simulink model "HILsim"  (R2024a)
settings: Solver=ode8  StartTime=0.0  StopTime=inf  FixedStep=SampleTime  RelTol=1e-3
values from neighbouring files (symbols this model uses):
  Arm = [ ... (first row only)    [launch.m]
  CDDrone = 0.01    [launch.m]
  CDval = 0.008    [launch.m]
  g = 9.81    [launch.m]
  m = 1.9    [launch.m]
  m_to_mm = 1000    [launch.m]
  ms_to_cms = 100    [launch.m]
  prop_inertia = (1/12) * 0.015 * 0.127^2    (= 2.016125e-05)    [launch.m]
  R = 0.127    [launch.m]
  ref_height = 76    [launch.m]
  ref_lat = 437818446e-7    (= 43.7818446)    [launch.m]
  ref_lon = -794679715e-7    (= -79.4679715)    [launch.m]
  rotorRPMMax = 10000    [launch.m]
  rotorTimeConst = 0.05    [launch.m]
  SampleTime = 0.004    [launch.m]
  tilt_speed = [0; pi/4; 0]    [launch.m]
  uT_to_gauss = 0.01    [launch.m]
undefined symbols (not defined in the file or in its folder): contact, control, ddx, ddy, ddz, dx, dy, dz, fractalcoef, lastVh, p, Payload, pitch, q, r, roll, X, Y, yaw, Z
libraries: uavmavlinklib x9, simulink x3, sharedutil x3, px4MAVLinkBridgelib x2, aerolibatmos2 x1, sensorgpslib x1, robotcorelib x1, mspsensorlib x1, shared6dof x1, simulink_extras x1, matrix_library x1
(part 2 of 2)

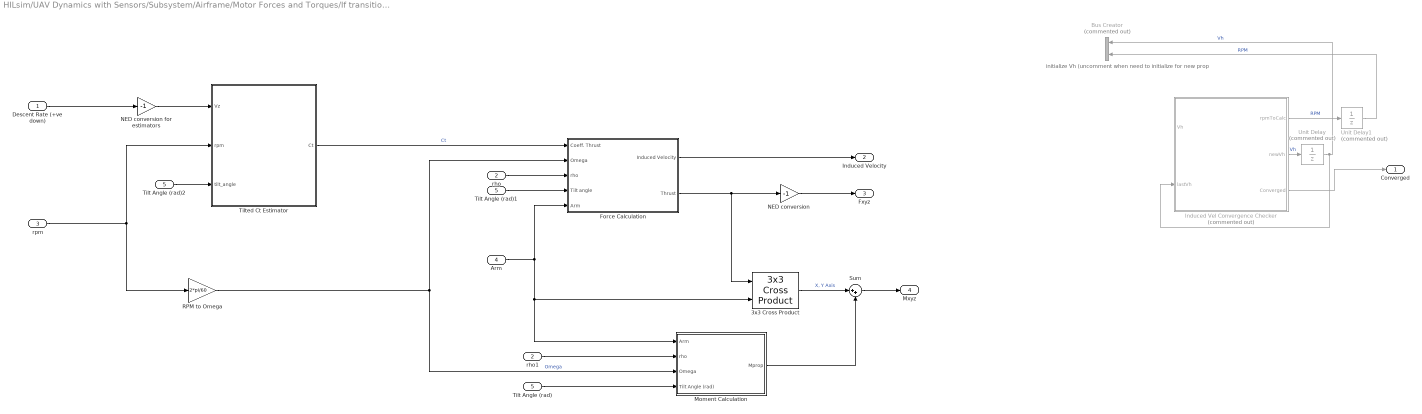
== system HILsim/UAV Dynamics with Sensors/Subsystem/Airframe/Motor Forces and Torques/If transitioning/Multirotor Subsystem/Rotor Subsystem ==
  note: initialize Vh (uncomment when need to initialize for new prop
  Descent Rate (+ve down) : Inport
  rho : Inport  Port=2
  rpm : Inport  Port=3
  Arm : Inport  Port=4
  Tilt Angle (rad) : Inport  Port=5
  3x3 Cross Product : sharedutil/3x3 Cross Product  aMode=aMode
      settings: LibrarySourceBlock=aerolibutil/3x3 Cross Product
  Bus Creator : BusCreator  Commented=on  Inputs=2
  Force Calculation : Subsystem
  Induced Vel Convergence Checker : MATLAB Function  Commented=on  TreatAsAtomicUnit=on  mask{VhInit=4.7, ConvThresh=1e-4}
      mask prompts: VhInit "Initial Vh Guess"; ConvThresh "Convergence Threshold"
  Moment Calculation : Subsystem
  NED conversion : Gain  Gain=-1
  NED conversion for estimators : Gain  Gain=-1
  RPM to Omega : Gain  Gain=2*pi/60
  Sum : Sum  Inputs=|++
  Tilt Angle (rad)1 : InportShadow  Port=5
  Tilt Angle (rad)2 : InportShadow  Port=5
  Tilted Ct Estimator : Subsystem
  Unit Delay : UnitDelay  Commented=on  InitialCondition=lastVh  SampleTime=0.001  HasFrameUpgradeWarning=on
  Unit Delay1 : UnitDelay  Commented=on  InitialCondition=1  SampleTime=0.001  HasFrameUpgradeWarning=on
  rho1 : InportShadow  Port=2
  Converged : Outport
  Induced Velocity : Outport  Port=2
  Fxyz : Outport  Port=3
  Mxyz : Outport  Port=4
  wires:
  Tilted Ct Estimator/1(Ct) -> Force Calculation/1(Coeff. Thrust)  "Ct"
  Unit Delay/1 -> Bus Creator/1, Induced Vel Convergence Checker/2(lastVh)  "Vh"
  Induced Vel Convergence Checker/3(Converged) -> Converged/1
  RPM to Omega/1 -> Moment Calculation/3(Omega), Force Calculation/2(Omega)  "Omega"
  rho/1 -> Force Calculation/3(rho)
  Induced Vel Convergence Checker/2(newVh) -> Unit Delay/1  "Vh"
  rpm/1 -> RPM to Omega/1, Tilted Ct Estimator/2(rpm)
  Descent Rate (+ve down)/1 -> NED conversion for estimators/1
  Unit Delay1/1 -> Bus Creator/2  "RPM"
  Induced Vel Convergence Checker/1(rpmToCalc) -> Unit Delay1/1  "RPM"
  Force Calculation/1(Induced Velocity) -> Induced Velocity/1
  Force Calculation/2(Thrust) -> NED conversion/1, 3x3 Cross Product/1
  3x3 Cross Product/1 -> Sum/1  "X, Y Axis"
  rho1/1 -> Moment Calculation/2(rho)
  Arm/1 -> 3x3 Cross Product/2, Moment Calculation/1(Arm), Force Calculation/5(Arm)
  Moment Calculation/1(Mprop) -> Sum/2
  Sum/1 -> Mxyz/1
  NED conversion/1 -> Fxyz/1
  Tilt Angle (rad)/1 -> Moment Calculation/4(Tilt Angle (rad))
  Tilt Angle (rad)1/1 -> Force Calculation/4(Tilt angle)
  NED conversion for estimators/1 -> Tilted Ct Estimator/1(Vz)
  Tilt Angle (rad)2/1 -> Tilted Ct Estimator/3(tilt_angle)

== system HILsim/UAV Dynamics with Sensors/Subsystem/Airframe/Motor Forces and Torques/If Tilted/Multirotor Subsystem/Rotor Subsystem/Ct Estimator ==
  note: this Vh curve is derived from performing a convergence
      | on the thrust curve
  note: Ct and Ct/Ct0 estimators are derived from CFD data
  Vz : Inport
  rpm : Inport  Port=2
  Abs : Abs  SaturateOnIntegerOverflow=off
  Calculate Ct : Product  Inputs=**
  Ct/C0 State Switcher : Subsystem
  Ct/Ct0 Estimator : Polyval  Coefs=[-0.012716815691322, -0.022830541813396, 0.156313447084851, -0.031641009616291, 1.004637965110952]
  Ct0 estimator for RPM : Polyval  Coefs=[0.000000000012185, -0.000000274732884, 0.008305365728125]
  Divide1 : Product  Inputs=*/
  NED conversion for estimators : Gain  Gain=-1
  Vh Calculator : Polyval  Coefs=[-5.17622414362771e-09, 0.000822973507549008, 0.0232660553338375]
  Ct : Outport
  wires:
  Abs/1 -> Ct0 estimator for RPM/1, Vh Calculator/1
  Divide1/1 -> Ct/Ct0 Estimator/1, Ct/C0 State Switcher/1(" Vz/Vh")  "Vz/Vh"
  Vh Calculator/1 -> Divide1/2  "Vh"
  Ct0 estimator for RPM/1 -> Calculate Ct/2  "Ct0"
  NED conversion for estimators/1 -> Divide1/1
  Ct/Ct0 Estimator/1 -> Ct/C0 State Switcher/2(Ct/C0 Fit)  "Ct/C0 Fit"
  Ct/C0 State Switcher/1(Out1) -> Calculate Ct/1  "Ct/C0"
  rpm/1 -> Abs/1
  Vz/1 -> NED conversion for estimators/1
  Calculate Ct/1 -> Ct/1  "Ct"

== system HILsim/UAV Dynamics with Sensors/Subsystem/Airframe/Motor Forces and Torques/If Tilted/Multirotor Subsystem/Rotor Subsystem/Force Calculation ==
  Coeff. Thrust : Inport
  Omega : Inport  Port=2
  rho : Inport  Port=3
  Arm : Inport  Port=4
  Constant : Constant  Value=0
  Divide : Product  Inputs=**
  Fx Sign : Subsystem
  Gain : Gain  Gain=cos(pi/4)
  Gain1 : Gain  Gain=sin(pi/4)
  Induced Vel Calc : Subsystem
  Math Function3 : Math  Operator=square  SignedPower=on
  Mux : Mux  Inputs=3
  Product6 : Product  Inputs=3
  R3 : Gain  Gain=R*R*pi*R*R
  Induced Velocity : Outport
  Thrust : Outport  Port=2
  wires:
  Math Function3/1 -> R3/1
  Induced Vel Calc/1(Vh) -> Induced Velocity/1
  R3/1 -> Product6/2
  Omega/1 -> Math Function3/1
  Gain1/1 -> Mux/3  "Fz"
  Constant/1 -> Mux/2  "Fy"
  Divide/1 -> Gain/1
  Product6/1 -> Divide/2, Gain1/1, Induced Vel Calc/1(Thrust)  "Fx"
  Fx Sign/1(Xsign) -> Divide/1
  Arm/1 -> Fx Sign/1(Arm)
  Gain/1 -> Mux/1  "Fx"
  Mux/1 -> Thrust/1
  Coeff. Thrust/1 -> Product6/3
  rho/1 -> Product6/1

== system HILsim/UAV Dynamics with Sensors/Subsystem/Airframe/Motor Forces and Torques/If Tilted/Multirotor Subsystem/Rotor Subsystem/Moment Calculation ==
  note: $\text{Torque about }z\text{ axis for the }i\text{th motor}: \frac{-1}{\sqrt2}(b\omega^2 + I_M \dot{w}), \text{where } b = \rho C_D AR^3$
  note: Angular Acceleration Term - $I_m \dot{\omega}$
  Arm : Inport
  rho : Inport  Port=2
  Omega : Inport  Port=3
  Abs : Abs  SaturateOnIntegerOverflow=off
  Divide : Product  Inputs=**
  Matrix Multiply : Product
  Moment of Inertia (1/12 m (a^2 + b^2)) : Gain  Gain=prop_inertia
  Mx Sign : Subsystem
  Mxy : Constant  Value=[0]
  OmegaDot : Derivative
  Product7 : Product
  R4 : Gain  Gain=CDval*R*R*R*pi*R*R
  Sum : Sum  Inputs=|++
  Vector Concatenate3 : Concatenate  NumInputs=3
  X : Gain  Gain=-1/sqrt(2)
  Z : Gain  Gain=-1/sqrt(2)
  Mprop : Outport
  wires:
  Vector Concatenate3/1 -> Mprop/1
  Omega/1 -> Abs/1, OmegaDot/1, Matrix Multiply/1
  OmegaDot/1 -> Moment of Inertia (1/12 m (a^2 + b^2))/1  "OmegaDot"
  Sum/1 -> Z/1, Divide/2
  Product7/1 -> Sum/1
  Moment of Inertia (1/12 m (a^2 + b^2))/1 -> Sum/2
  Z/1 -> Vector Concatenate3/3
  Divide/1 -> X/1
  Mxy/1 -> Vector Concatenate3/2  "Y"
  X/1 -> Vector Concatenate3/1
  Arm/1 -> Mx Sign/1(Arm)
  Mx Sign/1(Xsign) -> Divide/1
  Matrix Multiply/1 -> R4/1
  Abs/1 -> Matrix Multiply/2
  rho/1 -> Product7/1
  R4/1 -> Product7/2

== system HILsim/UAV Dynamics with Sensors/Subsystem/Airframe/Motor Forces and Torques/If non tilted/Multirotor Subsystem/Rotor Subsystem/Force Calculation ==
  Coeff. Thrust : Inport
  Omega : Inport  Port=2
  rho : Inport  Port=3
  Constant : Constant  Value=[0;0]  VectorParams1D=off
  Induced Vel Calc : Subsystem
  Math Function3 : Math  Operator=square  SignedPower=on
  Product6 : Product  Inputs=3
  R3 : Gain  Gain=R*R*pi*R*R
  Vector Concatenate : Concatenate
  Induced Velocity : Outport
  Thrust : Outport  Port=2
  wires:
  Coeff. Thrust/1 -> Product6/1
  Math Function3/1 -> R3/1
  Induced Vel Calc/1(Vh) -> Induced Velocity/1
  R3/1 -> Product6/2
  rho/1 -> Product6/3
  Omega/1 -> Math Function3/1
  Product6/1 -> Vector Concatenate/2, Induced Vel Calc/1(Thrust)  "Fz"
  Vector Concatenate/1 -> Thrust/1
  Constant/1 -> Vector Concatenate/1

== system HILsim/UAV Dynamics with Sensors/Subsystem/Airframe/Motor Forces and Torques/If non tilted/Multirotor Subsystem/Rotor Subsystem/Moment Calculation ==
  note: $\text{Torque about }z\text{ axis for the }i\text{th motor}: \frac{-1}{\sqrt2}(b\omega^2 + I_M \dot{w}), \text{where } b = \rho C_D AR^3$
  note: Angular Acceleration Term - $I_m \dot{\omega}$
  rho : Inport
  Omega : Inport  Port=2
  Abs : Abs  SaturateOnIntegerOverflow=off
  Matrix Multiply : Product
  Moment of Inertia (1/12 m (a^2 + b^2)) : Gain  Gain=prop_inertia
  Mxy : Constant  Value=[0;0]  VectorParams1D=off
  OmegaDot : Derivative
  Product7 : Product
  R4 : Gain  Gain=CDval*R*R*R*pi*R*R
  Sum : Sum  Inputs=|++
  Vector Concatenate3 : Concatenate
  Z : Gain  Gain=-1/sqrt(2)
  Mprop : Outport
  wires:
  Vector Concatenate3/1 -> Mprop/1
  R4/1 -> Product7/2
  rho/1 -> Product7/1
  Omega/1 -> Abs/1, OmegaDot/1, Matrix Multiply/1
  OmegaDot/1 -> Moment of Inertia (1/12 m (a^2 + b^2))/1  "OmegaDot"
  Sum/1 -> Z/1
  Product7/1 -> Sum/1
  Moment of Inertia (1/12 m (a^2 + b^2))/1 -> Sum/2
  Z/1 -> Vector Concatenate3/2
  Matrix Multiply/1 -> R4/1
  Abs/1 -> Matrix Multiply/2
  Mxy/1 -> Vector Concatenate3/1  "XY"

== system HILsim/UAV Dynamics with Sensors/Subsystem/Airframe/Motor Forces and Torques/If non tilted/Multirotor Subsystem/Rotor Subsystem/Non Tilted Ct estimator ==
  Vz : Inport
  RPM : Inport  Port=2
  Abs : Abs  SaturateOnIntegerOverflow=off
  Calculate Ct : Product  Inputs=**
  Ct/C0 State Switcher : Subsystem
  Ct/Ct0 Non Tilted Estimator : Polyval  Coefs=[0.147117704259973, 0.135195473604728, -0.341999514591595, -0.246799876690693, 0.999678014049876]
  Ct0 estimator for RPM : Polyval  Coefs=[0.000000000012185, -0.000000274732884, 0.008305365728125]
  Divide1 : Product  Inputs=*/
  Vh Calculator : Polyval  Coefs=[-5.17622414362771e-09, 0.000822973507549008, 0.0232660553338375]
  Ct : Outport
  wires:
  Abs/1 -> Vh Calculator/1, Ct0 estimator for RPM/1
  Calculate Ct/1 -> Ct/1  "Ct"
  Divide1/1 -> Ct/Ct0 Non Tilted Estimator/1, Ct/C0 State Switcher/1(" Vz/Vh")  "Vz/Vh"
  RPM/1 -> Abs/1
  Vh Calculator/1 -> Divide1/2  "Vh"
  Ct0 estimator for RPM/1 -> Calculate Ct/2  "Ct0"
  Ct/Ct0 Non Tilted Estimator/1 -> Ct/C0 State Switcher/2(Ct/C0 Fit)  "Ct/C0 Fit"
  Vz/1 -> Divide1/1
  Ct/C0 State Switcher/1(Ct/Ct0) -> Calculate Ct/1

== system HILsim/UAV Dynamics with Sensors/Subsystem/Airframe/Motor Forces and Torques/If transitioning/Multirotor Subsystem/Rotor Subsystem/Force Calculation ==
  Coeff. Thrust : Inport
  Omega : Inport  Port=2
  rho : Inport  Port=3
  Tilt angle : Inport  Port=4
  Arm : Inport  Port=5
  Components : Subsystem
  Fx Sign : Subsystem
  Induced Vel Calc : Subsystem
  Math Function3 : Math  Operator=square  SignedPower=on
  Mux : Mux  Inputs=3
  Product6 : Product  Inputs=3
  R3 : Gain  Gain=R*R*pi*R*R
  Induced Velocity : Outport
  Thrust : Outport  Port=2
  wires:
  Coeff. Thrust/1 -> Product6/1
  Math Function3/1 -> R3/1
  Induced Vel Calc/1(Vh) -> Induced Velocity/1
  R3/1 -> Product6/2
  rho/1 -> Product6/3
  Omega/1 -> Math Function3/1
  Product6/1 -> Components/3(F), Induced Vel Calc/1(Thrust)  "F"
  Arm/1 -> Fx Sign/1(Arm)
  Mux/1 -> Thrust/1
  Fx Sign/1(Xsign) -> Components/1(Sign)
  Tilt angle/1 -> Components/2(Tilt angle)
  Components/1(Fx) -> Mux/1
  Components/2(Fy) -> Mux/2
  Components/3(Fz) -> Mux/3

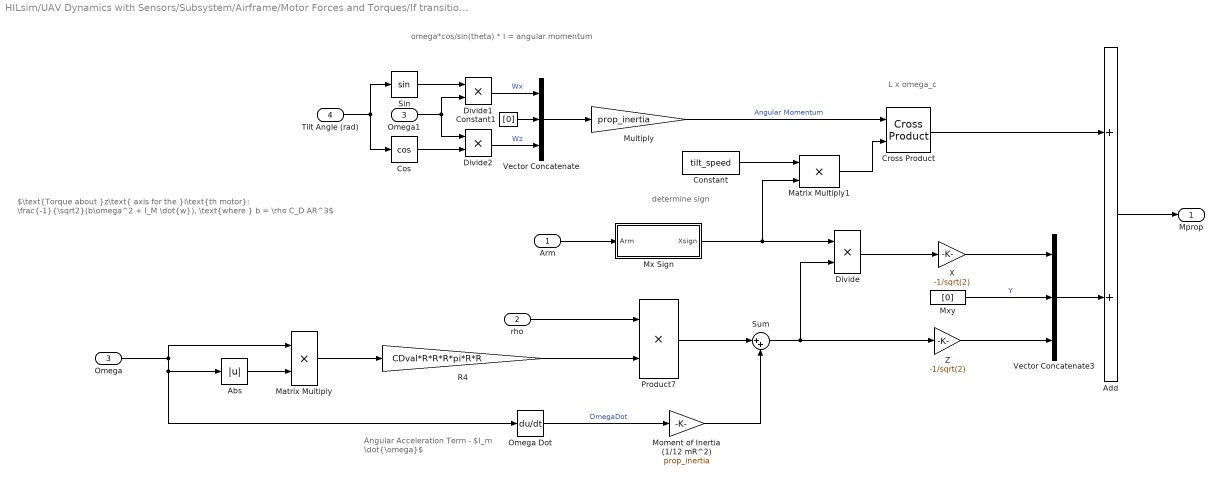
== system HILsim/UAV Dynamics with Sensors/Subsystem/Airframe/Motor Forces and Torques/If transitioning/Multirotor Subsystem/Rotor Subsystem/Moment Calculation ==
  note: determine sign
  note: L x omega_c
  note: omega*cos/sin(theta) * I = angular momentum
  note: $\text{Torque about }z\text{ axis for the }i\text{th motor}: \frac{-1}{\sqrt2}(b\omega^2 + I_M \dot{w}), \text{where } b = \rho C_D AR^3$
  note: Angular Acceleration Term - $I_m \dot{\omega}$
  Arm : Inport
  rho : Inport  Port=2
  Omega : Inport  Port=3
  Tilt Angle (rad) : Inport  Port=4
  Abs : Abs  SaturateOnIntegerOverflow=off
  Add : Sum
  Constant : Constant  Value=tilt_speed
  Constant1 : Constant  Value=[0]
  Cos : Trigonometry  Operator=cos
  Cross Product : matrix_library/Cross Product
  Divide : Product  Inputs=**
  Divide1 : Product  Inputs=**
  Divide2 : Product  Inputs=**
  Matrix Multiply : Product
  Matrix Multiply1 : Product
  Moment of Inertia (1/12 mR^2) : Gain  Gain=prop_inertia
  Multiply : Gain  Gain=prop_inertia
  Mx Sign : Subsystem
  Mxy : Constant  Value=[0]
  Omega Dot : Derivative
  Omega1 : InportShadow  Port=3
  Product7 : Product
  R4 : Gain  Gain=CDval*R*R*R*pi*R*R
  Sin : Trigonometry
  Sum : Sum  Inputs=|++
  Vector Concatenate : Concatenate  NumInputs=3
  Vector Concatenate3 : Concatenate  NumInputs=3
  X : Gain  Gain=-1/sqrt(2)
  Z : Gain  Gain=-1/sqrt(2)
  Mprop : Outport
  wires:
  R4/1 -> Product7/2
  rho/1 -> Product7/1
  Omega/1 -> Omega Dot/1, Abs/1, Matrix Multiply/1
  Omega Dot/1 -> Moment of Inertia (1/12 mR^2)/1  "OmegaDot"
  Sum/1 -> Z/1, Divide/2
  Product7/1 -> Sum/1
  Moment of Inertia (1/12 mR^2)/1 -> Sum/2
  Z/1 -> Vector Concatenate3/3
  Divide/1 -> X/1
  Mxy/1 -> Vector Concatenate3/2  "Y"
  Arm/1 -> Mx Sign/1(Arm)
  Mx Sign/1(Xsign) -> Divide/1, Matrix Multiply1/2
  Matrix Multiply/1 -> R4/1
  Abs/1 -> Matrix Multiply/2
  Tilt Angle (rad)/1 -> Cos/1, Sin/1
  Cos/1 -> Divide2/2
  Sin/1 -> Divide1/1
  Divide1/1 -> Vector Concatenate/1  "Wx"
  Vector Concatenate/1 -> Multiply/1
  Multiply/1 -> Cross Product/1  "Angular Momentum"
  Cross Product/1 -> Add/1
  Divide2/1 -> Vector Concatenate/3  "Wz"
  Constant1/1 -> Vector Concatenate/2
  Omega1/1 -> Divide2/1, Divide1/2
  Matrix Multiply1/1 -> Cross Product/2
  Constant/1 -> Matrix Multiply1/1
  X/1 -> Vector Concatenate3/1
  Vector Concatenate3/1 -> Add/2
  Add/1 -> Mprop/1

== system HILsim/UAV Dynamics with Sensors/Subsystem/Airframe/Motor Forces and Torques/If transitioning/Multirotor Subsystem/Rotor Subsystem/Tilted Ct Estimator ==
  note: - calculate ct/c0 from both estimators
      | - use tilt angle to perform a weighted average
  note: Accurate method:
      |
      | - model the tilt in ansys and find the thrust variation
  note: Possible simplified method:
      |
      | - stick to vrs dynamics from non tilted state for transitioning part -> more conservative
      | - do some interpolation between tilted and non tilted estimators
  Vz : Inport
  rpm : Inport  Port=2
  tilt_angle : Inport  Port=3
  Abs : Abs  SaturateOnIntegerOverflow=off
  Calculate Ct : Product  Inputs=**
  Ct/C0 State Switcher : Subsystem
  Ct0 estimator for RPM : Polyval  Coefs=[0.000000000012185, -0.000000274732884, 0.008305365728125]
  Divide1 : Product  Inputs=*/
  Vh Calculator : Polyval  Coefs=[-5.17622414362771e-09, 0.000822973507549008, 0.0232660553338375]
  Weighted Average Ct/C0 Fit : Subsystem
  Ct : Outport
  wires:
  Vh Calculator/1 -> Divide1/2  "Vh"
  Ct/C0 State Switcher/1(Out1) -> Calculate Ct/1  "Ct/C0"
  Divide1/1 -> Ct/C0 State Switcher/1(" Vz/Vh"), Weighted Average Ct/C0 Fit/1(Vz/Vh)  "Vz/Vh"
  rpm/1 -> Abs/1
  Abs/1 -> Vh Calculator/1, Ct0 estimator for RPM/1
  Ct0 estimator for RPM/1 -> Calculate Ct/2  "Ct0"
  Vz/1 -> Divide1/1
  Calculate Ct/1 -> Ct/1  "Ct"
  tilt_angle/1 -> Weighted Average Ct/C0 Fit/2(tilt_angle)
  Weighted Average Ct/C0 Fit/1(Out1) -> Ct/C0 State Switcher/2(Ct/C0 Fit)

== system HILsim/UAV Dynamics with Sensors/Subsystem/Airframe/Motor Forces and Torques/If Tilted/Multirotor Subsystem/Rotor Subsystem/Ct Estimator/Ct//C0 State Switcher ==
  " Vz/Vh" : Inport
  Ct/C0 Fit : Inport  Port=2
  " Vz/Vh1" : InportShadow
  Constant : Constant  Value=1.00463796511
  If : If  IfExpression=u1 >= -2.828427125 & u1 <= 0  ElseIfExpressions=u1 < -2.828427125
  If Action Subsystem : Subsystem  TreatAsAtomicUnit=on
  If Action Subsystem1 : Subsystem  TreatAsAtomicUnit=on
  If Action Subsystem2 : Subsystem  TreatAsAtomicUnit=on
  Merge : Merge  Inputs=3
  Scope1 : Scope
  Out1 : Outport
  wires:
  If Action Subsystem2/1(Out1) -> Merge/3
  If/3 -> If Action Subsystem2/Action  "climb"
  If/1 -> If Action Subsystem/Action  "descent"
  If Action Subsystem/1(Out1) -> Merge/1
  " Vz/Vh"/1 -> If/1
  If/2 -> If Action Subsystem1/Action  "past curve fit"
  Merge/1 -> Scope1/1, Out1/1
  Ct/C0 Fit/1 -> If Action Subsystem/1(In1)
  Constant/1 -> If Action Subsystem2/1("  ")
  If Action Subsystem1/1(" ") -> Merge/2
  " Vz/Vh1"/1 -> If Action Subsystem1/1(" Vz/Vh")

== system HILsim/UAV Dynamics with Sensors/Subsystem/Airframe/Motor Forces and Torques/If Tilted/Multirotor Subsystem/Rotor Subsystem/Force Calculation/Fx Sign ==
  Arm : Inport
  Sign : Signum
  X selector : Selector  InputPortWidth=3  IndexOptions=Index vector (dialog)  Indices=[1]  OutputSizes=1
  Xsign : Outport
  wires:
  Arm/1 -> X selector/1
  X selector/1 -> Sign/1
  Sign/1 -> Xsign/1

== system HILsim/UAV Dynamics with Sensors/Subsystem/Airframe/Motor Forces and Torques/If Tilted/Multirotor Subsystem/Rotor Subsystem/Force Calculation/Induced Vel Calc ==
  Thrust : Inport
  Denom : Constant  Value=2*1.225*pi*R^2
  Divide : Product  Inputs=*/
  Sqrt : Sqrt  OutDataTypeStr=double
  Vh : Outport
  wires:
  Denom/1 -> Divide/2
  Divide/1 -> Sqrt/1
  Sqrt/1 -> Vh/1
  Thrust/1 -> Divide/1

== system HILsim/UAV Dynamics with Sensors/Subsystem/Airframe/Motor Forces and Torques/If Tilted/Multirotor Subsystem/Rotor Subsystem/Moment Calculation/Mx Sign ==
  Arm : Inport
  Sign : Signum
  X selector : Selector  InputPortWidth=3  IndexOptions=Index vector (dialog)  Indices=[1]  OutputSizes=1
  Xsign : Outport
  wires:
  Arm/1 -> X selector/1
  X selector/1 -> Sign/1
  Sign/1 -> Xsign/1

== system HILsim/UAV Dynamics with Sensors/Subsystem/Airframe/Motor Forces and Torques/If non tilted/Multirotor Subsystem/Rotor Subsystem/Force Calculation/Induced Vel Calc ==
  Thrust : Inport
  Denom : Constant  Value=2*1.225*pi*R^2
  Divide : Product  Inputs=*/
  Saturation : Saturate  UpperLimit=inf  LowerLimit=0
  Sqrt : Sqrt  OutDataTypeStr=double
  Vh : Outport
  wires:
  Denom/1 -> Divide/2
  Divide/1 -> Saturation/1
  Sqrt/1 -> Vh/1
  Thrust/1 -> Divide/1
  Saturation/1 -> Sqrt/1

== system HILsim/UAV Dynamics with Sensors/Subsystem/Airframe/Motor Forces and Torques/If non tilted/Multirotor Subsystem/Rotor Subsystem/Non Tilted Ct estimator/Ct//C0 State Switcher ==
  note: add random number variations to VRS thrust to simulate thrust fluctuations
  " Vz/Vh" : Inport
  Ct/C0 Fit : Inport  Port=2
  " Vz/Vh1" : InportShadow
  Climb : Subsystem  TreatAsAtomicUnit=on
  Constant : Constant  Value=0.9905
  Descent : Subsystem  TreatAsAtomicUnit=on
  If : If  IfExpression=u1 >= -2 & u1 <= 0  ElseIfExpressions=u1 < -2
  Merge : Merge  Inputs=3
  Past Curve Fit : Subsystem  TreatAsAtomicUnit=on
  Ct/Ct0 : Outport
  wires:
  Past Curve Fit/1(" ") -> Merge/2
  Climb/1(Out1) -> Merge/3
  If/3 -> Climb/Action
  If/1 -> Descent/Action
  If/2 -> Past Curve Fit/Action
  Ct/C0 Fit/1 -> Descent/1(In1)
  " Vz/Vh1"/1 -> Past Curve Fit/1(" Vz/Vh")
  Constant/1 -> Climb/1("  ")
  Merge/1 -> Ct/Ct0/1
  Descent/1(Out1) -> Merge/1
  " Vz/Vh"/1 -> If/1

== system HILsim/UAV Dynamics with Sensors/Subsystem/Airframe/Motor Forces and Torques/If transitioning/Multirotor Subsystem/Rotor Subsystem/Force Calculation/Components ==
  Sign : Inport
  Tilt angle : Inport  Port=2
  F : Inport  Port=3
  Constant : Constant  Value=0
  Cos : Trigonometry
  Divide : Product  Inputs=**
  Matrix Multiply : Product
  Matrix Multiply1 : Product
  Sin : Trigonometry  Operator=cos
  Fx : Outport
  Fy : Outport  Port=2
  Fz : Outport  Port=3
  wires:
  Tilt angle/1 -> Cos/1, Sin/1
  Sign/1 -> Divide/1
  Sin/1 -> Matrix Multiply1/1
  Constant/1 -> Fy/1  "Fy"
  Cos/1 -> Matrix Multiply/2
  Matrix Multiply/1 -> Fx/1  "Fx"
  Divide/1 -> Matrix Multiply/1
  F/1 -> Matrix Multiply1/2, Divide/2
  Matrix Multiply1/1 -> Fz/1  "Fz"

== system HILsim/UAV Dynamics with Sensors/Subsystem/Airframe/Motor Forces and Torques/If transitioning/Multirotor Subsystem/Rotor Subsystem/Force Calculation/Fx Sign ==
  Arm : Inport
  Sign : Signum
  X selector : Selector  InputPortWidth=3  IndexOptions=Index vector (dialog)  Indices=[1]  OutputSizes=1
  Xsign : Outport
  wires:
  Arm/1 -> X selector/1
  X selector/1 -> Sign/1
  Sign/1 -> Xsign/1

== system HILsim/UAV Dynamics with Sensors/Subsystem/Airframe/Motor Forces and Torques/If transitioning/Multirotor Subsystem/Rotor Subsystem/Force Calculation/Induced Vel Calc ==
  Thrust : Inport
  Denom : Constant  Value=2*1.225*pi*R^2
  Divide : Product  Inputs=*/
  Sqrt : Sqrt  OutDataTypeStr=double
  Vh : Outport
  wires:
  Denom/1 -> Divide/2
  Divide/1 -> Sqrt/1
  Sqrt/1 -> Vh/1
  Thrust/1 -> Divide/1

== system HILsim/UAV Dynamics with Sensors/Subsystem/Airframe/Motor Forces and Torques/If transitioning/Multirotor Subsystem/Rotor Subsystem/Moment Calculation/Mx Sign ==
  Arm : Inport
  Sign : Signum
  X selector : Selector  InputPortWidth=3  IndexOptions=Index vector (dialog)  Indices=[1]  OutputSizes=1
  Xsign : Outport
  wires:
  Arm/1 -> X selector/1
  X selector/1 -> Sign/1
  Sign/1 -> Xsign/1

== system HILsim/UAV Dynamics with Sensors/Subsystem/Airframe/Motor Forces and Torques/If transitioning/Multirotor Subsystem/Rotor Subsystem/Tilted Ct Estimator/Ct//C0 State Switcher ==
  " Vz/Vh" : Inport
  Ct/C0 Fit : Inport  Port=2
  " Vz/Vh1" : InportShadow
  Constant : Constant  Value=1.00463796511
  If : If  IfExpression=u1 >= -2.828427125 & u1 <= 0  ElseIfExpressions=u1 < -2.828427125
  If Action Subsystem : Subsystem  TreatAsAtomicUnit=on
  If Action Subsystem1 : Subsystem  TreatAsAtomicUnit=on
  If Action Subsystem2 : Subsystem  TreatAsAtomicUnit=on
  Merge : Merge  Inputs=3
  Out1 : Outport
  wires:
  If Action Subsystem1/1(" ") -> Merge/2
  If Action Subsystem2/1(Out1) -> Merge/3
  If/3 -> If Action Subsystem2/Action  "climb"
  If/1 -> If Action Subsystem/Action  "descent"
  If Action Subsystem/1(Out1) -> Merge/1
  " Vz/Vh"/1 -> If/1
  If/2 -> If Action Subsystem1/Action  "past curve fit"
  Merge/1 -> Out1/1
  Ct/C0 Fit/1 -> If Action Subsystem/1(In1)
  " Vz/Vh1"/1 -> If Action Subsystem1/1(" Vz/Vh")
  Constant/1 -> If Action Subsystem2/1("  ")

== system HILsim/UAV Dynamics with Sensors/Subsystem/Airframe/Motor Forces and Torques/If transitioning/Multirotor Subsystem/Rotor Subsystem/Tilted Ct Estimator/Weighted Average Ct//C0 Fit ==
  Vz/Vh : Inport
  tilt_angle : Inport  Port=2
  Add : Sum
  Constant1 : Constant  Value=pi/4
  Constant2 : Constant
  Ct/Ct0 Non Tilted Estimator : Polyval  Coefs=[0.147117704259973, 0.135195473604728, -0.341999514591595, -0.246799876690693, 0.999678014049876]
  Ct/Ct0 Tilted Estimator : Polyval  Coefs=[-0.012716815691322, -0.022830541813396, 0.156313447084851, -0.031641009616291, 1.004637965110952]
  Divide1 : Product  Inputs=*/
  Matrix Multiply : Product
  Matrix Multiply1 : Product
  Subtract : Sum  Inputs=+-
  Out1 : Outport
  wires:
  Ct/Ct0 Tilted Estimator/1 -> Matrix Multiply/1  "Ct/C0 Fit"
  Vz/Vh/1 -> Ct/Ct0 Non Tilted Estimator/1, Ct/Ct0 Tilted Estimator/1
  Matrix Multiply/1 -> Add/1
  Ct/Ct0 Non Tilted Estimator/1 -> Matrix Multiply1/2  "Ct/C0 Fit"
  Matrix Multiply1/1 -> Add/2
  tilt_angle/1 -> Divide1/1
  Divide1/1 -> Matrix Multiply/2, Subtract/2
  Constant1/1 -> Divide1/2
  Constant2/1 -> Subtract/1
  Subtract/1 -> Matrix Multiply1/1
  Add/1 -> Out1/1

== system HILsim/UAV Dynamics with Sensors/Subsystem/Airframe/Motor Forces and Torques/If Tilted/Multirotor Subsystem/Rotor Subsystem/Ct Estimator/Ct//C0 State Switcher/If Action Subsystem ==
  In1 : Inport
  Action Port : ActionPort  ActionPortLabel=if(u1 >= -2.828427125 & u1 <= 0)
  Out1 : Outport
  wires:
  In1/1 -> Out1/1

== system HILsim/UAV Dynamics with Sensors/Subsystem/Airframe/Motor Forces and Torques/If Tilted/Multirotor Subsystem/Rotor Subsystem/Ct Estimator/Ct//C0 State Switcher/If Action Subsystem1 ==
  note: 1/2 * ln(-(x+1.23626605195)) + 1.814813688
  " Vz/Vh" : Inport
  Action Port : ActionPort  ActionPortLabel=elseif(u1 < -2.828427125)
  Add : Sum
  Constant : Constant  Value=1.814813688
  Constant1 : Constant  Value=1.23626605195
  Gain : Gain  Gain=1/2
  Multiply : Gain  Gain=-1
  Saturation : Saturate  UpperLimit=inf  LowerLimit=0.001
  Sum : Sum  Inputs=|++
  ln : Math  Operator=log
  " " : Outport
  wires:
  Gain/1 -> Add/1
  Constant/1 -> Add/2
  " Vz/Vh"/1 -> Sum/1
  Sum/1 -> Multiply/1
  Constant1/1 -> Sum/2
  Add/1 -> " "/1
  Multiply/1 -> Saturation/1
  ln/1 -> Gain/1
  Saturation/1 -> ln/1

== system HILsim/UAV Dynamics with Sensors/Subsystem/Airframe/Motor Forces and Torques/If Tilted/Multirotor Subsystem/Rotor Subsystem/Ct Estimator/Ct//C0 State Switcher/If Action Subsystem2 ==
  "  " : Inport
  Action Port : ActionPort  ActionPortLabel=else
  Out1 : Outport
  wires:
  "  "/1 -> Out1/1

== system HILsim/UAV Dynamics with Sensors/Subsystem/Airframe/Motor Forces and Torques/If non tilted/Multirotor Subsystem/Rotor Subsystem/Non Tilted Ct estimator/Ct//C0 State Switcher/Climb ==
  "  " : Inport
  Action Port : ActionPort  ActionPortLabel=else
  Out1 : Outport
  wires:
  "  "/1 -> Out1/1

== system HILsim/UAV Dynamics with Sensors/Subsystem/Airframe/Motor Forces and Torques/If non tilted/Multirotor Subsystem/Rotor Subsystem/Non Tilted Ct estimator/Ct//C0 State Switcher/Descent ==
  In1 : Inport
  Action Port : ActionPort  ActionPortLabel=if(u1 >= -2 & u1 <= 0)
  Out1 : Outport
  wires:
  In1/1 -> Out1/1

== system HILsim/UAV Dynamics with Sensors/Subsystem/Airframe/Motor Forces and Torques/If non tilted/Multirotor Subsystem/Rotor Subsystem/Non Tilted Ct estimator/Ct//C0 State Switcher/Past Curve Fit ==
  note: 1/2*ln(-(x+1.7439783573836165)) + 2.07884583669
  " Vz/Vh" : Inport
  Action Port : ActionPort  ActionPortLabel=elseif(u1 < -2)
  Add : Sum
  Constant : Constant  Value=2.07884583669
  Constant1 : Constant  Value=1.7439783573836165
  Gain : Gain  Gain=1/2
  Multiply : Gain  Gain=-1
  Saturation : Saturate  UpperLimit=inf  LowerLimit=0.0001
  Sum : Sum  Inputs=|++
  ln : Math  Operator=log
  " " : Outport
  wires:
  Add/1 -> " "/1
  Constant/1 -> Add/2
  Multiply/1 -> Saturation/1
  ln/1 -> Gain/1
  " Vz/Vh"/1 -> Sum/1
  Sum/1 -> Multiply/1
  Constant1/1 -> Sum/2
  Gain/1 -> Add/1
  Saturation/1 -> ln/1

== system HILsim/UAV Dynamics with Sensors/Subsystem/Airframe/Motor Forces and Torques/If transitioning/Multirotor Subsystem/Rotor Subsystem/Tilted Ct Estimator/Ct//C0 State Switcher/If Action Subsystem ==
  In1 : Inport
  Action Port : ActionPort  ActionPortLabel=if(u1 >= -2.828427125 & u1 <= 0)
  Out1 : Outport
  wires:
  In1/1 -> Out1/1

== system HILsim/UAV Dynamics with Sensors/Subsystem/Airframe/Motor Forces and Torques/If transitioning/Multirotor Subsystem/Rotor Subsystem/Tilted Ct Estimator/Ct//C0 State Switcher/If Action Subsystem1 ==
  " Vz/Vh" : Inport
  Action Port : ActionPort  ActionPortLabel=elseif(u1 < -2.828427125)
  Add : Sum
  Constant : Constant  Value=1.007639046
  Multiply : Gain  Gain=-1
  ln : Math  Operator=log
  " " : Outport
  wires:
  Add/1 -> " "/1
  Constant/1 -> Add/2
  Multiply/1 -> ln/1
  " Vz/Vh"/1 -> Multiply/1
  ln/1 -> Add/1

== system HILsim/UAV Dynamics with Sensors/Subsystem/Airframe/Motor Forces and Torques/If transitioning/Multirotor Subsystem/Rotor Subsystem/Tilted Ct Estimator/Ct//C0 State Switcher/If Action Subsystem2 ==
  "  " : Inport
  Action Port : ActionPort  ActionPortLabel=else
  Out1 : Outport
  wires:
  "  "/1 -> Out1/1

== matlab function HILsim/UAV Dynamics with Sensors/Subsystem/Airframe/Motor Forces and Torques/If transitioning/Multirotor Subsystem/Rotor Subsystem/Induced Vel Convergence Checker ==
  data: rpmToCalc output; newVh output; Converged output; Vh input; convergence_threshold parameter; lastVh input
function [rpmToCalc, newVh, Converged] = CalculateInducedVelocity(Vh, convergence_threshold, lastVh)

    % Initialize variables
    persistent rpm_index rpm_values Vh_values exportedCoefficients;

    if isempty(rpm_index)
        rpm_index = 1;
        rpm_values = 1:1000:10001;
        Vh_values = zeros(size(rpm_values));
        exportedCoefficients = false;
    end

    if rpm_index > 11
        rpmToCalc = 1;
        newVh = 0.1;
        Converged = 1;
        return;
    end

    % Calculate the difference between the current and last induced velocity
    difference = abs(Vh - lastVh);
    rpmToCalc = rpm_values(rpm_index);

    if difference < convergence_threshold
        % Convergence achieved
        Converged = 1;
        newVh = Vh; % Update to the current induced velocity
        Vh_values(rpm_index) = Vh;
        
        if rpm_index >= length(rpm_values) && exportedCoefficients == false
            coefficients = fitVhToRPM(rpm_values, Vh_values);
            assignin('base', 'coefficients', coefficients);
            assignin('base', 'rpm_values', rpm_values);
            assignin('base', 'Vh_values', Vh_values);
            exportedCoefficients = true;
            return;
        else
            if rpm_index ~= 11
                rpmToCalc = rpm_values(rpm_index+1);
            end
        end

        % Move to the next RPM value
        if rpm_index < 11
            rpm_index = rpm_index + 1;
        end
    else
        % Convergence not achieved
        Converged = 0;
        newVh = Vh; % Update to the new induced velocity
    end
end

function coefficients = fitVhToRPM(rpm_values, Vh_values)
    % Fit a polynomial (or any other function) to the RPM and Vh values
    p = polyfit(rpm_values, Vh_values, 2);
    coefficients = p;
end

== matlab function HILsim/UAV Dynamics with Sensors/Subsystem/Airframe/Motor Forces and Torques/If non tilted/Multirotor Subsystem/Rotor Subsystem/Induced Vel Convergence Checker ==
  data: rpmToCalc output; newVh output; Converged output; Vh input; convergence_threshold parameter; lastVh input
function [rpmToCalc, newVh, Converged] = CalculateInducedVelocity(Vh, convergence_threshold, lastVh)

    % Initialize variables
    persistent rpm_index rpm_values Vh_values exportedCoefficients;

    if isempty(rpm_index)
        rpm_index = 1;
        rpm_values = 1:1000:10001;
        Vh_values = zeros(size(rpm_values));
        exportedCoefficients = false;
    end

    if rpm_index > 11
        rpmToCalc = 1;
        newVh = 0.1;
        Converged = 1;
        return;
    end

    % Calculate the difference between the current and last induced velocity
    difference = abs(Vh - lastVh);
    rpmToCalc = rpm_values(rpm_index);

    if difference < convergence_threshold
        % Convergence achieved
        Converged = 1;
        newVh = Vh; % Update to the current induced velocity
        Vh_values(rpm_index) = Vh;
        
        if rpm_index >= length(rpm_values) && exportedCoefficients == false
            coefficients = fitVhToRPM(rpm_values, Vh_values);
            assignin('base', 'coefficients', coefficients);
            assignin('base', 'rpm_values', rpm_values);
            assignin('base', 'Vh_values', Vh_values);
            exportedCoefficients = true;
            return;
        else
            if rpm_index ~= 11
                rpmToCalc = rpm_values(rpm_index+1);
            end
        end

        % Move to the next RPM value
        if rpm_index < 11
            rpm_index = rpm_index + 1;
        end
    else
        % Convergence not achieved
        Converged = 0;
        newVh = Vh; % Update to the new induced velocity
    end
end

function coefficients = fitVhToRPM(rpm_values, Vh_values)
    % Fit a polynomial (or any other function) to the RPM and Vh values
    p = polyfit(rpm_values, Vh_values, 2);
    coefficients = p;
end

== matlab function HILsim/UAV Dynamics with Sensors/Subsystem/Airframe/Motor Forces and Torques/If Tilted/Multirotor Subsystem/Rotor Subsystem/Induced Vel Convergence Checker ==
  data: rpmToCalc output; newVh output; Converged output; Vh input; convergence_threshold parameter; lastVh input
function [rpmToCalc, newVh, Converged] = CalculateInducedVelocity(Vh, convergence_threshold, lastVh)

    % Initialize variables
    persistent rpm_index rpm_values Vh_values exportedCoefficients;

    if isempty(rpm_index)
        rpm_index = 1;
        rpm_values = 1:1000:10001;
        Vh_values = zeros(size(rpm_values));
        exportedCoefficients = false;
    end

    if rpm_index > 11
        rpmToCalc = 1;
        newVh = 0.1;
        Converged = 1;
        return;
    end

    % Calculate the difference between the current and last induced velocity
    difference = abs(Vh - lastVh);
    rpmToCalc = rpm_values(rpm_index);

    if difference < convergence_threshold
        % Convergence achieved
        Converged = 1;
        newVh = Vh; % Update to the current induced velocity
        Vh_values(rpm_index) = Vh;
        
        if rpm_index >= length(rpm_values) && exportedCoefficients == false
            coefficients = fitVhToRPM(rpm_values, Vh_values);
            assignin('base', 'coefficients', coefficients);
            assignin('base', 'rpm_values', rpm_values);
            assignin('base', 'Vh_values', Vh_values);
            exportedCoefficients = true;
            return;
        else
            if rpm_index ~= 11
                rpmToCalc = rpm_values(rpm_index+1);
            end
        end

        % Move to the next RPM value
        if rpm_index < 11
            rpm_index = rpm_index + 1;
        end
    else
        % Convergence not achieved
        Converged = 0;
        newVh = Vh; % Update to the new induced velocity
    end
end

function coefficients = fitVhToRPM(rpm_values, Vh_values)
    % Fit a polynomial (or any other function) to the RPM and Vh values
    p = polyfit(rpm_values, Vh_values, 2);
    coefficients = p;
end
